simulink model "Lab03_03_02"  (R2023a)
settings: Solver=VariableStepAuto  StartTime=0.0  StopTime=3  RelTol=1e-3
values from neighbouring files (symbols this model uses):
  den1 = [1 100000 2128000]    [Lab03.m]
  den2_2 = tf2.Denominator    [Lab03.m]
  dt1 = 0.00031999999192    [Señal1.mat]
  num1 = 2128000    [Lab03.m]
  num2_2 = tf2.Numerator    [Lab03.m]
settings Model: Creator=Daniela  LastModifiedBy=Daniela

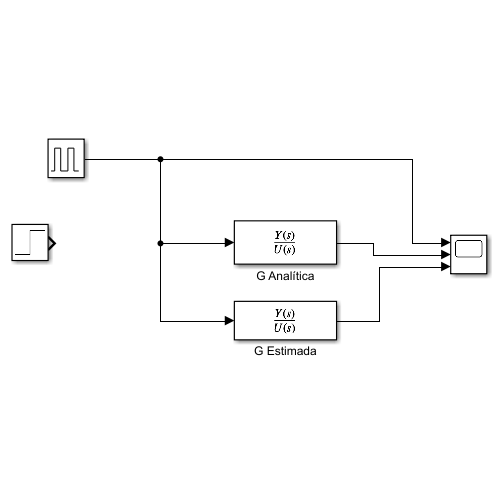
[thumbnail: Simulink's stored preview of the top-level diagram]
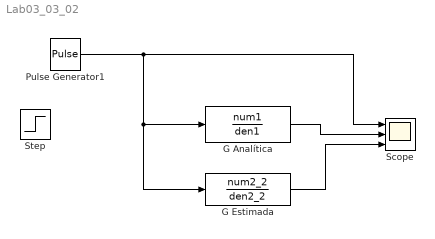
== system Lab03_03_02 ==
  G Analítica : TransferFcn  Numerator=num1  Denominator=den1
  G Estimada : TransferFcn  Numerator=num2_2  Denominator=den2_2
  Pulse Generator1 : DiscretePulseGenerator  PulseType=Time based  Amplitude=5  Period=3/2  PulseWidth=50
  Scope : Scope  NumInputPorts=3
  Step : Step  Time=0.015  After=5  SampleTime=dt1
  wires:
  G Analítica/1 -> Scope/2
  G Estimada/1 -> Scope/3
  Pulse Generator1/1 -> Scope/1, G Analítica/1, G Estimada/1
